simulink library "C_Block"  (R2019a)
settings: Solver=VariableStepAuto  StartTime=0.0  StopTime=10.0  RelTol=1e-3
settings Model: Creator=agmotes  LastModifiedBy=agmotes

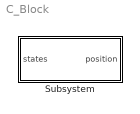
== system C_Block ==
  Subsystem : Subsystem

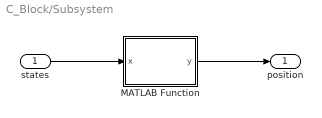
== system C_Block/Subsystem ==
  states : Inport
  MATLAB Function : MATLAB Function  TreatAsAtomicUnit=on
  position : Outport
  wires:
  states/1 -> MATLAB Function/1(x)
  MATLAB Function/1(y) -> position/1

== matlab function C_Block/Subsystem/MATLAB Function ==
  data: x input; y output
function y = C_Block(x)

y = x(1);
